simulink model "Lidar_System_August5"  (Simulink 7.3)
settings: Solver=FixedStepDiscrete  StartTime=0.0  StopTime=inf  FixedStep=0.1  MaxStep=0.2  RelTol=1e-3
libraries: dspmtrx3 x3, simulink x2, vipstatistics x1, dspstat3 x1
settings Model: Creator=gclayton  LastModifiedBy=wildcat
settings DebuggingCC: InheritedTsInSrcMsg=none
settings RTWCC: SystemTargetFile=rlnx.tlc  GenCodeOnly=on  TemplateMakefile=rlnx_ubuntu.tmf  Description=Linux Real-Time Target  ProcessScript=rlnx_make_rtw_hook
settings RTWCC: CustomInclude=|
  | /usr/local/include/opencv/
  | /usr/local/include/
settings CodeAppCC: GenerateComments=off  SimulinkBlockComments=off
settings STFCustomTargetCC: ModelReferenceCompliant=off  MatFileLogging=on  SystemTargetFile=rlnx.tlc
settings GRTTargetCC: ModelReferenceCompliant=off  ParMdlRefBuildCompliant=off  CompOptLevelCompliant=off
settings CustomProperty: DataType=string  Value="-lm -ldl /usr/local/lib/libopencv_highgui.so.2.4 /usr/local/lib/libopencv_core.so.2.4 /usr/local/lib/libopencv_imgproc.so.2.4  -lc_urg -lc_urg_connection -lc_urg_system -lphidget21 -llcm /matlab_includes/simulink/include/RXState_RXState_t.so /matlab_includes/simulink/include/fau_coordinate_t.so"
settings EnumStrPairs: String=PC

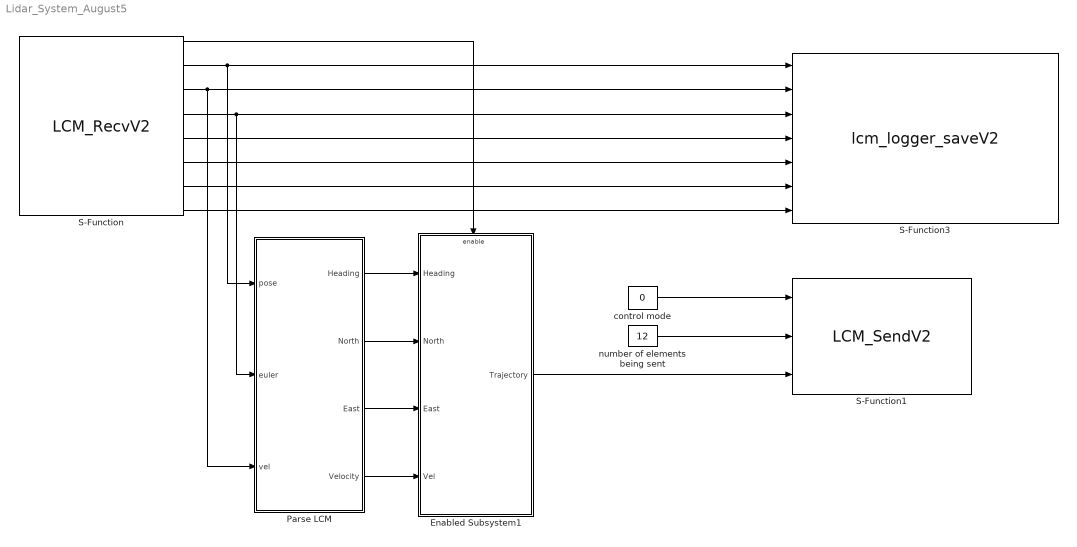
== system Lidar_System_August5 ==
  Enabled Subsystem1 : Subsystem  TreatAsAtomicUnit=on
  Parse LCM : Stateflow chart
  S-Function : S-Function  FunctionName=LCM_RecvV2  EnableBusSupport=off
      mask Display:
      | port_label('output',1,'enable')
      | port_label('output',2,'pose')
      | port_label('output',3,'vel')
      | port_label('output',4,'euler')
      | port_label('output',5,'portstate')
      | port_label('output',6,'stbdstate')
      | port_label('output',7,'starttime')
      | port_label('output',8,'elapsedtime')
      | 
      | fprintf('LCM_RecvV2')
  S-Function1 : S-Function  FunctionName=LCM_SendV2  EnableBusSupport=off
      mask Display:
      | port_label('input',1,'cmode')
      | port_label('input',2,'count')
      | port_label('input',3,'traject')
      | 
      | fprintf('LCM_SendV2')
  S-Function3 : S-Function  FunctionName=lcm_logger_saveV2  EnableBusSupport=off
  control mode : Constant  Value=0  OutDataTypeMode=int16  OutDataType=fixdt(1, 16)  OutScaling=2^0  OutDataTypeStr=int16
  number of elements being sent : Constant  Value=12  OutDataTypeMode=int16  OutDataType=fixdt(1, 16)  OutScaling=2^0  OutDataTypeStr=int16
  wires:
  S-Function/1 -> Enabled Subsystem1/Enable
  S-Function/2 -> Parse LCM/1(pose), S-Function3/1
  S-Function/3 -> S-Function3/2, Parse LCM/3(vel)
  S-Function/4 -> S-Function3/3, Parse LCM/2(euler)
  S-Function/5 -> S-Function3/4
  S-Function/6 -> S-Function3/5
  S-Function/7 -> S-Function3/6
  S-Function/8 -> S-Function3/7
  number of elements being sent/1 -> S-Function1/2
  Parse LCM/2(North) -> Enabled Subsystem1/2(North)
  control mode/1 -> S-Function1/1
  Enabled Subsystem1/1(Trajectory) -> S-Function1/3
  Parse LCM/3(East) -> Enabled Subsystem1/3(East)
  Parse LCM/1(Heading) -> Enabled Subsystem1/1(Heading)
  Parse LCM/4(Velocity) -> Enabled Subsystem1/4(Vel)

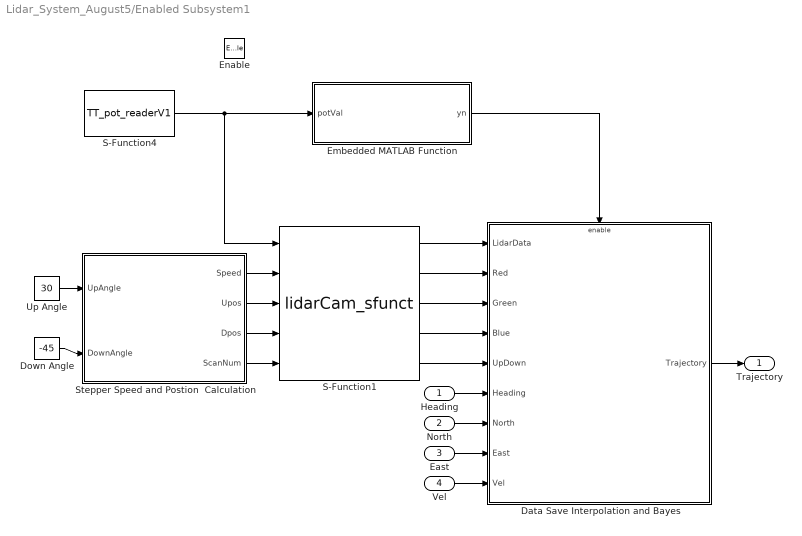
== system Lidar_System_August5/Enabled Subsystem1 ==
  Heading : Inport  OutDataType=fixdt(1, 16)  OutScaling=2^0
  North : Inport  Port=2  OutDataType=fixdt(1, 16)  OutScaling=2^0
  East : Inport  Port=3  OutDataType=fixdt(1, 16)  OutScaling=2^0
  Vel : Inport  Port=4  OutDataType=fixdt(1, 16)  OutScaling=2^0
  Enable : EnablePort
  Data Save Interpolation and Bayes : Subsystem  TreatAsAtomicUnit=on
  Down Angle : Constant  Value=-45  OutDataType=fixdt(1, 16)  OutScaling=2^0
  Embedded MATLAB Function : Stateflow chart
  S-Function1 : S-Function  FunctionName=lidarCam_sfunct  EnableBusSupport=off
  S-Function4 : S-Function  FunctionName=TT_pot_readerV1  EnableBusSupport=off
  Stepper Speed and Postion  Calculation : Stateflow chart
  Up Angle : Constant  Value=30  OutDataType=fixdt(1, 16)  OutScaling=2^0
  Trajectory : Outport  OutDataType=fixdt(1, 16)  OutScaling=2^0
  wires:
  S-Function4/1 -> S-Function1/1, Embedded MATLAB Function/1(potVal)
  Stepper Speed and Postion  Calculation/1(Speed) -> S-Function1/2
  Stepper Speed and Postion  Calculation/2(Upos) -> S-Function1/3
  Stepper Speed and Postion  Calculation/3(Dpos) -> S-Function1/4
  Stepper Speed and Postion  Calculation/4(ScanNum) -> S-Function1/5
  Embedded MATLAB Function/1(yn) -> Data Save Interpolation and Bayes/Enable
  S-Function1/1 -> Data Save Interpolation and Bayes/1(LidarData)
  Down Angle/1 -> Stepper Speed and Postion  Calculation/2(DownAngle)
  Up Angle/1 -> Stepper Speed and Postion  Calculation/1(UpAngle)
  S-Function1/5 -> Data Save Interpolation and Bayes/5(UpDown)
  S-Function1/2 -> Data Save Interpolation and Bayes/2(Red)
  S-Function1/3 -> Data Save Interpolation and Bayes/3(Green)
  S-Function1/4 -> Data Save Interpolation and Bayes/4(Blue)
  Heading/1 -> Data Save Interpolation and Bayes/6(Heading)
  North/1 -> Data Save Interpolation and Bayes/7(North)
  East/1 -> Data Save Interpolation and Bayes/8(East)
  Data Save Interpolation and Bayes/1(Trajectory) -> Trajectory/1
  Vel/1 -> Data Save Interpolation and Bayes/9(Vel)

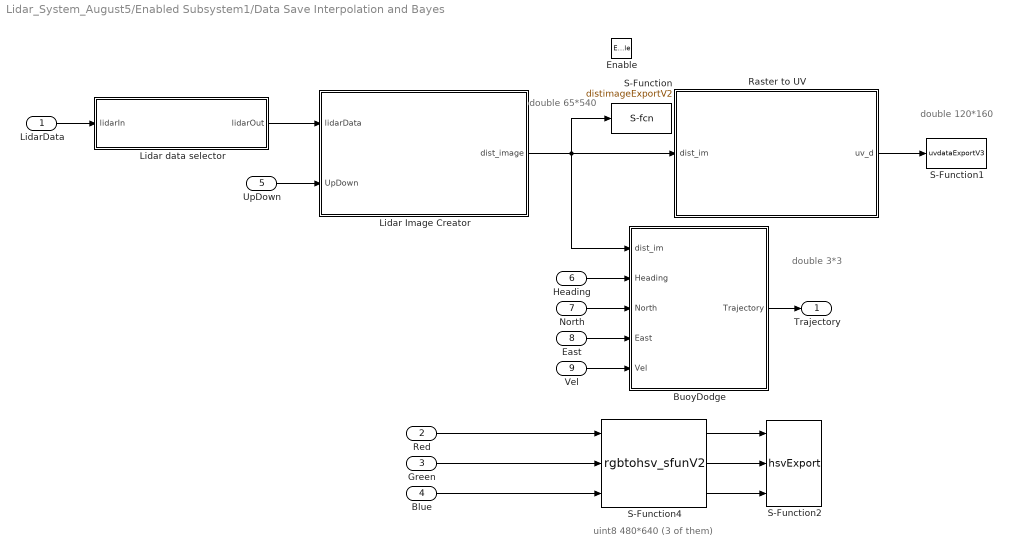
== system Lidar_System_August5/Enabled Subsystem1/Data Save Interpolation and Bayes ==
  note: uint8 480*640 (3 of them)
  note: double 120*160
  note: double 65*540
  note: double 3*3
  LidarData : Inport  OutDataType=fixdt(1, 16)  OutScaling=2^0
  Red : Inport  Port=2  OutDataType=fixdt(1, 16)  OutScaling=2^0
  Green : Inport  Port=3  OutDataType=fixdt(1, 16)  OutScaling=2^0
  Blue : Inport  Port=4  OutDataType=fixdt(1, 16)  OutScaling=2^0
  UpDown : Inport  Port=5  OutDataType=fixdt(1, 16)  OutScaling=2^0
  Heading : Inport  Port=6  OutDataType=fixdt(1, 16)  OutScaling=2^0
  North : Inport  Port=7  OutDataType=fixdt(1, 16)  OutScaling=2^0
  East : Inport  Port=8  OutDataType=fixdt(1, 16)  OutScaling=2^0
  Vel : Inport  Port=9  OutDataType=fixdt(1, 16)  OutScaling=2^0
  Enable : EnablePort
  BuoyDodge : Subsystem
  Lidar Image Creator : Stateflow chart
  Lidar data selector : Stateflow chart
  Raster to UV : Stateflow chart
  S-Function : S-Function  FunctionName=distimageExportV2  EnableBusSupport=off
  S-Function1 : S-Function  FunctionName=uvdataExportV3  EnableBusSupport=off
  S-Function2 : S-Function  FunctionName=hsvExport  EnableBusSupport=off
  S-Function4 : S-Function  FunctionName=rgbtohsv_sfunV2  EnableBusSupport=off
  Trajectory : Outport  OutDataType=fixdt(1, 16)  OutScaling=2^0
  wires:
  Lidar data selector/1(lidarOut) -> Lidar Image Creator/1(lidarData)
  UpDown/1 -> Lidar Image Creator/2(UpDown)
  Lidar Image Creator/1(dist_image) -> BuoyDodge/1(dist_im), Raster to UV/1(dist_im), S-Function/1
  Red/1 -> S-Function4/1
  Green/1 -> S-Function4/2
  Blue/1 -> S-Function4/3
  LidarData/1 -> Lidar data selector/1(lidarIn)
  BuoyDodge/1(Trajectory) -> Trajectory/1
  Heading/1 -> BuoyDodge/2(Heading)
  North/1 -> BuoyDodge/3(North)
  East/1 -> BuoyDodge/4(East)
  S-Function4/1 -> S-Function2/1
  S-Function4/2 -> S-Function2/2
  S-Function4/3 -> S-Function2/3
  Raster to UV/1(uv_d) -> S-Function1/1
  Vel/1 -> BuoyDodge/5(Vel)

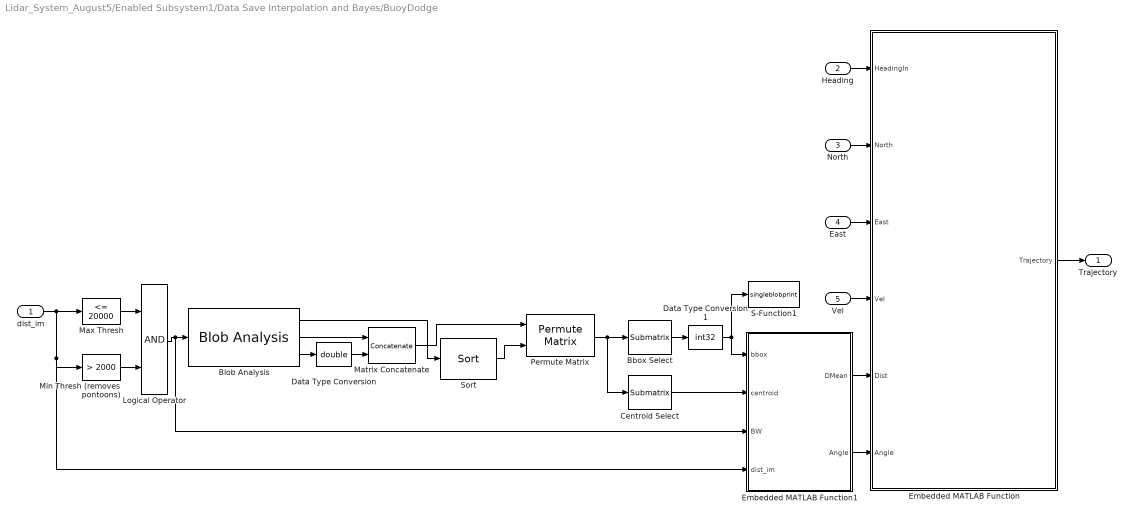
== system Lidar_System_August5/Enabled Subsystem1/Data Save Interpolation and Bayes/BuoyDodge ==
  dist_im : Inport  OutDataType=fixdt(1, 16)  OutScaling=2^0
  Heading : Inport  Port=2  OutDataType=fixdt(1, 16)  OutScaling=2^0
  North : Inport  Port=3  OutDataType=fixdt(1, 16)  OutScaling=2^0
  East : Inport  Port=4  OutDataType=fixdt(1, 16)  OutScaling=2^0
  Vel : Inport  Port=5  OutDataType=fixdt(1, 16)  OutScaling=2^0
  Bbox Select : dspmtrx3/Submatrix  RowSpan=Range of rows  RowStartMode=Index  RowStartIndex=3  RowEndMode=Last  RowEndIndex=4  ColSpan=One column  ColStartMode=First  ColStartIndex=1  ColEndMode=Last  ColEndIndex=1
  Blob Analysis : vipstatistics/Blob Analysis  DialogController=vipDDGCreate  DialogControllerArgs=DataTag0  area=on  centroid=on  bBox=on  majorAxis=off  minorAxis=off  angle=off  eccentricity=off  equivDiameterSq=off  extent=off  perimeter=off  maxBlobs=12  warnIfNumBlobsExceeded=on  isCount=off  useMinArea=off  minArea=0  useMaxArea=off  maxArea=intmax('uint32')  excludeBorderBlob=off  outDT=double  isOutVarDim=off  isFill=on  fillValues=-1  conn=8  isLabel=off  outputMode=Binary point scaling  outputWordLength=32  outputFracLength=16  firstCoeffMode=Binary point scaling  firstCoeffWordLength=16  firstCoeffFracLength=14  secondCoeffMode=Binary point scaling  secondCoeffWordLength=32  secondCoeffFracLength=16  accumMode=Binary point scaling  accumWordLength=32  accumFracLength=0  prodOutputMode=Binary point scaling  prodOutputWordLength=32  prodOutputFracLength=16  roundingMode=Floor  overflowMode=off
  Centroid Select : dspmtrx3/Submatrix  RowSpan=Range of rows  RowStartMode=First  RowStartIndex=5  RowEndMode=Index  RowEndIndex=2  ColSpan=One column  ColStartMode=First  ColStartIndex=1  ColEndMode=Last  ColEndIndex=1
  Data Type Conversion : DataTypeConversion  OutDataTypeMode=double  OutDataType=fixdt(1, 16)  OutScaling=2^0  OutDataTypeStr=double
  Data Type Conversion1 : DataTypeConversion  OutDataTypeMode=int32  OutDataType=fixdt(1, 16)  OutScaling=2^0  OutDataTypeStr=int32
  Embedded MATLAB Function : Stateflow chart
  Embedded MATLAB Function1 : Stateflow chart
  Logical Operator : Logic  AllPortsSameDT=off  OutDataTypeMode=boolean  LogicDataType=fixdt(0, 8)  OutDataTypeStr=boolean
  Matrix Concatenate : Concatenate  Mode=Multidimensional array
  Max Thresh : simulink/Logic and Bit Operations/Compare To Constant  SystemSampleTime=-1  relop=<=  const=20000  LogicOutDataTypeMode=boolean  ZeroCross=off
  Min Thresh (removes pontoons) : simulink/Logic and Bit Operations/Compare To Constant  SystemSampleTime=-1  relop=>  const=2000  LogicOutDataTypeMode=boolean  ZeroCross=off
  Permute Matrix : dspmtrx3/Permute Matrix  mode=Columns  ZeroOneIdxMode=One-based  errmode=Clip index  checkDims=off
  S-Function1 : S-Function  FunctionName=singleblobprint  EnableBusSupport=off
  Sort : dspstat3/Sort  DialogController=dspDDGCreate  DialogControllerArgs=DataTag1  otype=Index  dir=Descending  sortAlg=Quick sort  roundingMode=Floor  overflowMode=off
  Trajectory : Outport  OutDataType=fixdt(1, 16)  OutScaling=2^0
  wires:
  dist_im/1 -> Max Thresh/1, Min Thresh (removes pontoons)/1, Embedded MATLAB Function1/4(dist_im)
  Max Thresh/1 -> Logical Operator/1
  Min Thresh (removes pontoons)/1 -> Logical Operator/2
  Logical Operator/1 -> Blob Analysis/1, Embedded MATLAB Function1/3(BW)
  Sort/1 -> Permute Matrix/2
  Permute Matrix/1 -> Bbox Select/1, Centroid Select/1
  Blob Analysis/2 -> Matrix Concatenate/1
  Blob Analysis/3 -> Data Type Conversion/1
  Matrix Concatenate/1 -> Permute Matrix/1
  Blob Analysis/1 -> Sort/1
  Bbox Select/1 -> Data Type Conversion1/1
  Centroid Select/1 -> Embedded MATLAB Function1/2(centroid)
  Embedded MATLAB Function/1(Trajectory) -> Trajectory/1
  Heading/1 -> Embedded MATLAB Function/1(HeadingIn)
  North/1 -> Embedded MATLAB Function/2(North)
  East/1 -> Embedded MATLAB Function/3(East)
  Data Type Conversion/1 -> Matrix Concatenate/2
  Embedded MATLAB Function1/1(DMean) -> Embedded MATLAB Function/5(Dist)
  Embedded MATLAB Function1/2(Angle) -> Embedded MATLAB Function/6(Angle)
  Data Type Conversion1/1 -> Embedded MATLAB Function1/1(bbox), S-Function1/1
  Vel/1 -> Embedded MATLAB Function/4(Vel)

== matlab function Parse LCM ==
  data: pose input double; Heading output double; euler input double; North output double; East output double; vel input double; Velocity output double
function [Heading, North, East, Velocity] = ParseLCM(pose,euler,vel)
%Written by Anderson Lebbad on July 22, 2014
%Last Edited:

%This function takes in the LCM read variables and parses for necessary
%information

Heading = euler(3);
North = pose(1);
East = pose(2);
Velocity = sqrt(vel(1)^2+vel(2)^2); 
end

== matlab function Enabled Subsystem1/Data Save Interpolation and Bayes/BuoyDodge/Embedded MATLAB Function ==
  data: HeadingIn input double; Trajectory output double; North input double; East input double; Vel input double; Dist input double; Angle input double
function Trajectory   = BuoyTrajectories( HeadingIn, North, East, Vel,...
    Dist, Angle )
%Written by Anderson Lebbad on July 21, 2014
%Last Edited: July 22, 2014 for NED coordinate system

%This function takes the distance and angle found to a single obstacle, and
%the current heading and GPS information to create a trajectory to dodge
%the buoy. If no buoy is found, the trajectory is set for a forward
%straight line motion

%Convert Heading to radians
Heading = HeadingIn*pi/180;

%Distance past buoy to set end point, further than length of boat
dodgeLength = 10;

%Distance to the side the boat dodges around the buoy
dodgeWidth = 10;

%Variable to track how many frames it has been since last trajectory has
%been output - don't send a new trajectory until first one is completed
persistent frames

if isempty(frames)
    frames = 0;
end

if frames >= 10
    frames = 0;
end

%Set size of output matrix
Trajectory = zeros(4,3);

if frames == 0
    %First trajectory point is starting point (current)
    North = North + 5*cos(Heading);
    East = East + 5*sin(Heading);
    Trajectory(1,:) = [North, East, 0];
    if Dist ~= 0
        %Calculate heading to found buoy
        BuoyHeading = (mod(Heading + Angle, 360))*pi/180;
        %Find an offset angle to dodge around buoy at same distance as buoy
        offsetAngle = dodgeWidth/Dist;
        %Find heading to that angle
        offsetHeading = BuoyHeading + offsetAngle;
        %Find the north and east coordinates to offset point
        offsetNorth = North + Dist*cos(offsetHeading);
        offsetEast = East + Dist*sin(offsetHeading);
        %Calculate time to get to first point
        offsetTime = 5*cos(Vel*pi/2)+ sqrt(Dist^2+dodgeWidth^2);
        %Second trajectory point is the offset point
        Trajectory(2,:) = [offsetNorth, offsetEast, offsetTime];
        %Calculate distance to end point
        endDist = Dist + dodgeLength;
        %Find the north and east coordinates to end point
        endNorth = North + endDist*cos(Heading);
        endEast = East + endDist*sin(Heading);
        %Calculate time to end point
        endTime = offsetTime + sqrt(dodgeWidth^2+dodgeLength^2);
        %Third trajectory point is the end point
        Trajectory(3,:) = [endNorth, endEast, endTime];
        frames = 1;
    else
        %If no buoy is found, go two lengths of the boat
        %Calculate GPS point to one length of the boat forward at current
        %heading
        %Find the latitude and longitude of the point
        oneNorth =  North + dodgeLength*cos(Heading);
        oneEast = East + dodgeLength*sin(Heading);
        %Calculate time to the point
        oneTime = 5*cos(Vel*pi/2) + Dist;
        %Second trajectory point is the one length away point
        Trajectory(2,:) = [oneNorth, oneEast, oneTime];
        %Calculate GPS point to two lengths of the boat forward at current
        %heading
        %Find the latitude and longitude of the point
        twoNorth =  North + 2*dodgeLength*cos(Heading);
        twoEast = East + 2*dodgeLength*sin(Heading);
        %Calculate time to the point
        twoTime = oneTime + Dist;
        %Second trajectory point is the one length away point
        Trajectory(3,:) = [twoNorth, twoEast, twoTime];
    end
    %Set a final point to straighten out and continue along original path
    finalNorth = Trajectory(3,1) + dodgeLength*cos(Heading);
    finalEast = Trajectory(3,2) + dodgeLength*sin(Heading);
    finalTime = Trajectory(3,3) + dodgeLength;
    Trajectory(4,:) = [finalNorth, finalEast, finalTime];
else
    frames = frames + 1;
end
        
end

== matlab function Enabled Subsystem1/Data Save Interpolation and Bayes/BuoyDodge/Embedded MATLAB Function1 ==
  data: bbox input double; centroid input double; BW input double; dist_im input double; DMean output double; Angle output double
function [DMean, Angle] = bbox_hist(bbox, centroid, BW, dist_im)
%Written by Anderson Lebbad on July 22, 2014
%Last Edited:

%This function finds the average depth of a detected blob and the relative
%angle of it

%Initialize variables
pixels = 0;
DRunAve = 0;

%Parse bbox data
left = bbox(2) + 1;
right = left + bbox(4) - 1;
bottom = bbox(1) + 1;
top = bottom + bbox(3) - 1;

%Calculate angle based off centroid. Dist_im has 540 horizontal columns
%that cover a 135 field of view (4 points per degree)
Angle = centroid(2)/4 - 67.5;

%Check to see if valid bbox is found
if left~=-1
    %Scan the detected region of the binary image and generate histograms
    for j=left:right
        for i=bottom:top
            if BW(i,j) == 1
                pixels = pixels + 1;
                DRunAve = ((pixels-1)/pixels)*DRunAve + (1/pixels)*double(dist_im(i,j));
            end
        end
    end
end

%Output meterss
DMean = DRunAve/1000;

end

== matlab function Enabled Subsystem1/Data Save Interpolation and Bayes/Raster to UV ==
  data: uv_d output double; dist_im input double
function uv_d   = AngleMatch( dist_im )
%Written by Anderson Lebbad on July 8, 2014
%Last Edited:

%This function infers depth locations into a image plane based upon the
%angles as they relate to the field of view of the camera. This works
%decently, but loses accuracy at closer ranges as the spacial translation
%between the video camera and lidar becomes more noticeable

%% Initialize

uv_d = zeros(120,160);

%% Parameters

%Camera field of view to determines indices to match
FoVx = 62;
FoVy = 46;

%Scan angles for lidar gimbal
upAngle = 30;
downAngle = -45;
angleRange = upAngle-downAngle;

%% Operation

% Depth frame, same aspect ratio as image frame, quarter width and height
for i = 1:160
    for j = 1:120
        % Effective coordinate in pixel frame
        u = (i-1)/(160-1)*(640-1)+1;
        v = (j-1)/(120-1)*(480-1)+1;
        
        % Scan angle for pixel location being analyzed in degrees
        scanAngleHoriz = -FoVx/2 + (u-1)*FoVx/(640-1);
        scanAngleVert = FoVy/2 - (v-1)*FoVy/(480-1) - 4;
        
        % Estimate closest scan value for pixel being evaluated
        xCenter = round((67.5+scanAngleHoriz)*(540-1)/135+1);
        yCenter = round((upAngle-scanAngleVert)*(65-1)/(angleRange)+1);
        
        % Assign
        uv_d(j,i) = dist_im(yCenter,xCenter);
    end
end

end

== matlab function Enabled Subsystem1/Data Save Interpolation and Bayes/Lidar Image Creator ==
  data: lidarData input double; dist_image output double; UpDown input double
function dist_image = scanImages(lidarData,UpDown)
%Written by Anderson Lebbad on July 5, 2014
%Last Edited:

%Converts the one dimensional array of lidarData and the scan settings into
%frames of distances and angles for each point

% Set output sizes
dist_image = zeros(65,540);

% To run through the middle half of the points horizonatal points, the
% first quarter must be skipped (of 1080)
scanOffset = 270-1;

% Loop through all points in output matrices
for j=1:540
    for i=1:65
        % Select the lidarData that will be used in analysis and format as
        % a frame
        dist_image(i,j) = lidarData(j+scanOffset+1080*(i-1));
    end
end

% Flip if up scan
if UpDown
    dist_image = flipud(dist_image);
end

dist_image = fliplr(dist_image);

end

== matlab function Enabled Subsystem1/Data Save Interpolation and Bayes/Lidar data selector ==
  data: lidarIn input double; lidarOut output double
function lidarOut = data_selector(lidarIn)
% Lidar data is always input as a 1x70200 matrix.
% If Scan Number is less than 65 some of this data may be blank
% Select only the parts of the matrix where data has been collected

FullLength = 1080*65;
DataLength =  1080*65;
lidarOut = zeros(FullLength,1);

% ClosePts = (lidarIn < 3);
% lidarOut = (lidarIn + 30000*ClosePts)/10;

for i = 1:DataLength
    if (lidarIn(i,1) < 3)
        lidarIn(i,1) = 30000;
    end
    lidarOut(i,1) = lidarIn(i,1);
end

%lidarOut = lidarIn(1,1:DataLength);

== matlab function Enabled Subsystem1/Embedded MATLAB Function ==
  data: potVal input double; yn output double
function yn = check_pot_val(potVal)
%#eml

% Pot value may initially be zero.
% Check for this and output a 1 or zero to 
% control whether the rest of model runs
if (potVal == 0)
    yn = 0;
else
    yn = 1;
end

== matlab function Enabled Subsystem1/Stepper Speed and Postion Calculation ==
  data: UpAngle input double; Speed output double; DownAngle input double; Upos output double; Dpos output double; ScanNum output double
function [Speed,Upos,Dpos,ScanNum] = stepper_calc(UpAngle,DownAngle)
% Last Edited by Anderson Lebbad on July 7, 2014
% edits were made to account for new calibration on gimbal

% This function inputs desired positive and negative scan angles
% and desired number of scans and outputs results positions for
% the stepper and the required speed of the stepper motor to properly
% move so the desired number of scans is obtained over the course of
% the motion of the stepper

% Scan Number requires no change
ScanNum = 65;
% Number of steps for 180 degree flip
stepRes = 3950;
% Parameter to account for slack in the gears with respect to steps
stepGive = 57;

% Transformation of angle to stepper position obtained from stepper calibration
% Output must be an integer
% 57 is added or subtracted due to wobble of gimbal system
Upos = round(UpAngle*stepRes/180)-stepGive;
Dpos = round(DownAngle*stepRes/180)+stepGive;

% Transformation of speed based 
% Output must be an interger
Speed = round(abs(UpAngle-DownAngle) * (1214/90));
